simulink model "abb_inv_dyn"  (R2023b)
settings: Solver=ode45  StartTime=0.0  StopTime=inf  RelTol=1e-3
undefined symbols (not defined in the file): abb_eom_solution, abbRobot, control_inv_dyn, hamiltonian_fun_solution, I_Je_fun_solution, I_r_IE_fun_solution
libraries: simulink x7
settings Model: Creator=dario  LastModifiedBy=slin
settings SolverCC: AlgebraicLoopSolver=TrustRegion
settings DataIOCC: LimitDataPoints=on  SaveFormat=Array  ReturnWorkspaceOutputs=off
settings OptimizationCC: BlockReduction=off  BooleanDataType=off  LifeSpan=inf
settings DebuggingCC: SaveWithParameterizedLinksMsg=none  UnderspecifiedInitializationDetection=Classic  MergeDetectMultiDrivingBlocksExec=none  SignalResolutionControl=TryResolveAllWithWarning  FcnCallInpInsideContextMsg=warning  UnconnectedInputMsg=warning  UnconnectedOutputMsg=warning  UnconnectedLineMsg=warning  SFUnexpectedBacktrackingDiag=warning  SFNoUnconditionalDefaultTransitionDiag=warning  ArithmeticOperatorsInVariantConditions=warning
settings HardwareCC: ProdBitPerPointer=32  ProdBitPerSizeT=32  ProdBitPerPtrDiffT=32  ProdLargestAtomicFloat=None  ProdIntDivRoundTo=Undefined  ProdEndianess=Unspecified  ProdWordSize=32  ProdHWDeviceType=32-bit Generic  TargetUnknown=on
settings ModelReferenceCC: EnableRefExpFcnMdlSchedulingChecks=on  PropagateSignalLabelsOutOfModel=off
settings SFSimCC: SimUseLocalCustomCode=off  CustomCodeUndefinedFunction=UseInterfaceOnly
settings RTWCC: RTWUseLocalCustomCode=off
settings CodeAppCC: StateflowObjectComments=on
settings GRTTargetCC: TargetLangStandard=C89/C90 (ANSI)
settings ConfigComp: CovMetricSettings=dw  CovSaveCumulativeToWorkspaceVar=on  CovSaveSingleToWorkspaceVar=on  CovExternalEMLEnable=off

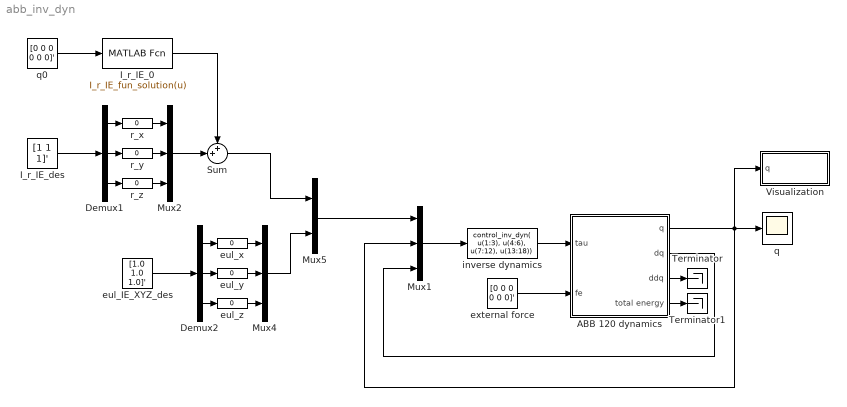
== system abb_inv_dyn ==
  ABB 120 dynamics : Subsystem  mask{Ts=0.01, F=[0.1 0.1 0.1 0.1 0.1 0.1]', phi0=[0 0 0 0 0 0]', dphi0=[0 0 0 0 0 0]', enable_g=on, enable_f=off}
      mask prompts: Ts "Sample time"; F "Viscous friction (6x1)"; phi0 "Initial joint positions"; dphi0 "Initial joint velocities"; enable_g "Enable gravity"; enable_f "Enable friction"
  Demux1 : Demux  Outputs=3
  Demux2 : Demux  Outputs=3
  I_r_IE_0 : MATLABFcn  MATLABFcn=I_r_IE_fun_solution(u)  OutputDimensions=[3,1]  Output1D=off
  I_r_IE_des : Constant  Value=[1 1 1]'
  Mux1 : Mux  Inputs=3
  Mux2 : Mux  Inputs=3
  Mux4 : Mux  Inputs=3
  Mux5 : Mux  Inputs=2
  Sum : Sum  Inputs=++|
  Terminator : Terminator
  Terminator1 : Terminator
  Visualization : Subsystem
  eul_IE_XYZ_des : Constant  Value=[1.0 1.0 1.0]'
  eul_x : simulink/Math Operations/Slider Gain  gain=0  low=-2  high=2
  eul_y : simulink/Math Operations/Slider Gain  gain=0  low=-2  high=2
  eul_z : simulink/Math Operations/Slider Gain  gain=0  low=-2  high=2
  external force : Constant  Value=[0 0 0 0 0 0]'
  inverse dynamics : MATLABFcn  MATLABFcn=control_inv_dyn( u(1:3), u(4:6), u(7:12), u(13:18))  OutputDimensions=[6,1]  Output1D=off
  q : Scope
  q0 : Constant  Value=[0 0 0 0 0 0]'
  r_x : simulink/Math Operations/Slider Gain  gain=0  low=-2  high=2
  r_y : simulink/Math Operations/Slider Gain  gain=0  low=-2  high=2
  r_z : simulink/Math Operations/Slider Gain  gain=0  low=-2  high=2
  wires:
  ABB 120 dynamics/1(q) -> q/1, Visualization/1(q), Mux1/2
  external force/1 -> ABB 120 dynamics/2(fe)
  Mux1/1 -> inverse dynamics/1
  ABB 120 dynamics/2(dq) -> Mux1/3
  inverse dynamics/1 -> ABB 120 dynamics/1(tau)
  ABB 120 dynamics/3(ddq) -> Terminator/1
  ABB 120 dynamics/4(total energy) -> Terminator1/1
  Mux5/1 -> Mux1/1
  Demux1/1 -> r_x/1
  Demux1/2 -> r_y/1
  r_z/1 -> Mux2/3
  r_y/1 -> Mux2/2
  r_x/1 -> Mux2/1
  Demux1/3 -> r_z/1
  I_r_IE_des/1 -> Demux1/1
  Demux2/1 -> eul_x/1
  Demux2/2 -> eul_y/1
  eul_z/1 -> Mux4/3
  eul_y/1 -> Mux4/2
  eul_x/1 -> Mux4/1
  Demux2/3 -> eul_z/1
  eul_IE_XYZ_des/1 -> Demux2/1
  Mux4/1 -> Mux5/2
  Sum/1 -> Mux5/1
  Mux2/1 -> Sum/2
  I_r_IE_0/1 -> Sum/1
  q0/1 -> I_r_IE_0/1

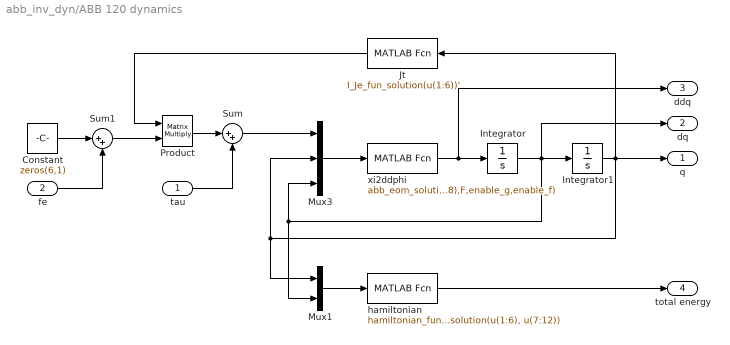
== system abb_inv_dyn/ABB 120 dynamics ==
  tau : Inport
  fe : Inport  Port=2
  Constant : Constant  Value=zeros(6,1)
  Integrator : Integrator  InitialCondition=dphi0
  Integrator1 : Integrator  InitialCondition=phi0
  Jt : MATLABFcn  MATLABFcn=I_Je_fun_solution(u(1:6))'  OutputDimensions=[6,6]  OutputSignalType=real  Output1D=off
  Mux1 : Mux  Inputs=2
  Mux3 : Mux  Inputs=3
  Product : Product  Multiplication=Matrix(*)
  Sum : Sum  Inputs=|++
  Sum1 : Sum  Inputs=|++
  hamiltonian : MATLABFcn  MATLABFcn=hamiltonian_fun_solution(u(1:6), u(7:12))  OutputDimensions=[1,1]  Output1D=off
  xi2ddphi : MATLABFcn  MATLABFcn=abb_eom_solution(u(1:6), u(7:12), u(13:18),F,enable_g,enable_f)  OutputDimensions=[6,1]  Output1D=off
  q : Outport
  dq : Outport  Port=2
  ddq : Outport  Port=3
  total energy : Outport  Port=4
  wires:
  Integrator/1 -> Mux1/2, Mux3/3, dq/1, Integrator1/1
  tau/1 -> Sum/2
  Integrator1/1 -> Jt/1, Mux1/1, Mux3/2, q/1
  Mux3/1 -> xi2ddphi/1
  xi2ddphi/1 -> ddq/1, Integrator/1
  Mux1/1 -> hamiltonian/1
  hamiltonian/1 -> total energy/1
  Jt/1 -> Product/1
  Product/1 -> Sum/1
  Sum/1 -> Mux3/1
  Constant/1 -> Sum1/1
  fe/1 -> Sum1/2
  Sum1/1 -> Product/2

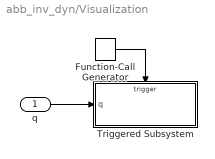
== system abb_inv_dyn/Visualization ==
  q : Inport
  Function-Call Generator : simulink/Ports & Subsystems/Function-Call Generator  sample_time=0.05  numberOfIterations=1  DisallowWideOutput=off
  Triggered Subsystem : Subsystem  TreatAsAtomicUnit=on
  wires:
  Function-Call Generator/1 -> Triggered Subsystem/Trigger
  q/1 -> Triggered Subsystem/1(q)

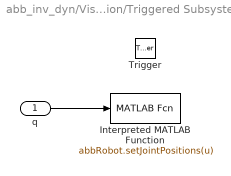
== system abb_inv_dyn/Visualization/Triggered Subsystem ==
  q : Inport
  Trigger : TriggerPort  TriggerType=function-call  VariantControl=Variant
  Interpreted MATLAB Function : MATLABFcn  MATLABFcn=abbRobot.setJointPositions(u)  OutputDimensions=0
  wires:
  q/1 -> Interpreted MATLAB Function/1
